simulink model "Fuzzy_PID_1"  (R2024a)
settings: Solver=VariableStepAuto  StartTime=0.0  StopTime=10.0  RelTol=1e-3
libraries: fuzblock x1
settings Model: Creator=Miko  LastModifiedBy=Miko

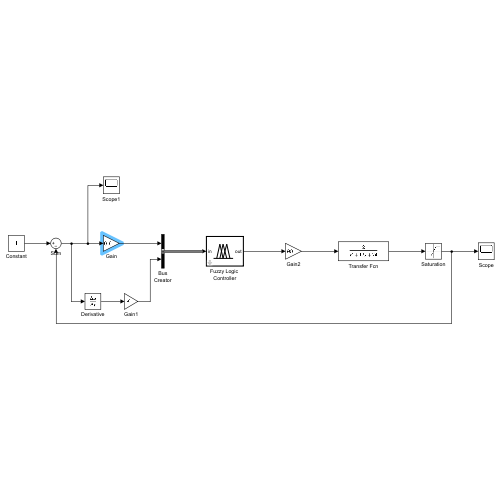
[thumbnail: Simulink's stored preview of the top-level diagram]
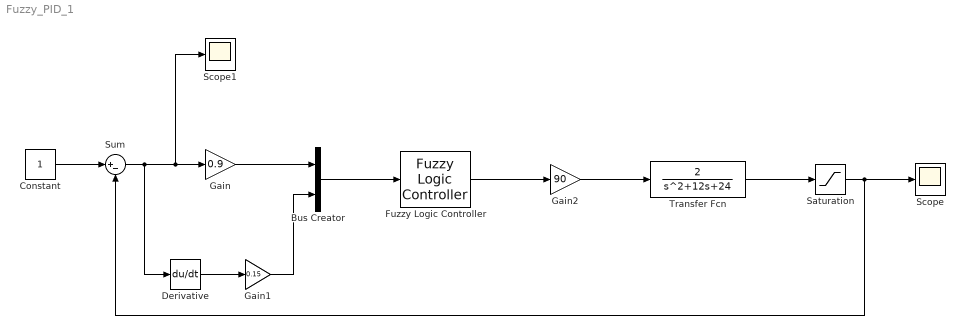
== system Fuzzy_PID_1 ==
  Bus Creator : BusCreator  Inputs=2
  Constant : Constant
  Derivative : Derivative
  Fuzzy Logic Controller : fuzblock/Fuzzy Logic  Controller  FIS='motorFIS.fis'  OutputSampleNumber=101  DataType=double  FuzzifiedInputs=off  RuleFiringStrengths=off  RuleOutputs=off  AggregatedOutputs=off  SimulateUsing=Interpreted execution  OutOfRangeInputValueMessage=warning  NoRuleFiredMessage=warning  EmptyOutputFuzzySetMessage=warning
  Gain : Gain  Gain=0.9
  Gain1 : Gain  Gain=0.15
  Gain2 : Gain  Gain=90
  Saturation : Saturate  UpperLimit=1  LowerLimit=-1
  Scope : Scope
  Scope1 : Scope
  Sum : Sum  Inputs=|+-
  Transfer Fcn : TransferFcn  Numerator=[2]  Denominator=[1 12 24]
  wires:
  Constant/1 -> Sum/1
  Sum/1 -> Derivative/1, Scope1/1, Gain/1
  Bus Creator/1 -> Fuzzy Logic Controller/1
  Gain/1 -> Bus Creator/1
  Derivative/1 -> Gain1/1
  Gain1/1 -> Bus Creator/2
  Fuzzy Logic Controller/1 -> Gain2/1
  Gain2/1 -> Transfer Fcn/1
  Transfer Fcn/1 -> Saturation/1
  Saturation/1 -> Sum/2, Scope/1
